simulink model "SWC_HALIN_type"  (R2021b)
settings: Solver=FixedStepDiscrete  StartTime=0.0  StopTime=10.0  FixedStep=0.005  RelTol=1e-3
undefined symbols (not defined in the file): FALSE, R_WDGCDD_CSOP_Call_Watchdog, R_WDGCDD_CSOP_Call_WDG_AppStart, TRUE
libraries: halin x1
settings Model: DataDictionary=APPTypes.sldd  Creator=FVT23010  LastModifiedBy=FVT23010
settings DataIOCC: SaveFormat=StructureWithTime
settings OptimizationCC: DefaultParameterBehavior=Inlined  EnhancedBackFolding=on  PassReuseOutputArgsAs=Individual arguments  ZeroExternalMemoryAtStartup=off  ZeroInternalMemoryAtStartup=off  OptimizeBlockOrder=speed  DifferentSizesBufferReuse=on  OptimizationCustomize=off  EfficientTunableParamExpr=on
settings DebuggingCC: ParameterTunabilityLossMsg=error
settings ModelReferenceCC: ModelReferenceNumInstancesAllowed=Single
settings SFSimCC: MATLABDynamicMemAlloc=off
settings RTWCC: Description=AUTOSAR  SystemTargetFile=autosar.tlc  GenCodeOnly=on  TemplateMakefile=ert_default_tmf
settings CodeAppCC: ForceParamTrailComments=on  IgnoreCustomStorageClasses=off  OperatorAnnotations=on  SimulinkDataObjDesc=on  SFDataObjDesc=on  InsertBlockDesc=on
settings STFCustomTargetCC: TargetLangStandard=C99 (ISO)  MultiwordLength=256  ParMdlRefBuildCompliant=on  CompOptLevelCompliant=on  IncludeMdlTerminateFcn=off  CombineOutputUpdateFcns=on  SuppressErrorStatus=on  ERTCustomFileBanners=on  SupportNonFinite=off  SupportComplex=off  SupportContinuousTime=off  SupportNonInlinedSFcns=off  RemoveResetFunc=on  MATLABClassNameForMDSCustomization=Simulink.SoftwareTarget.ERTCustomization  AutosarCompliant=on  GRTInterface=off  UseToolchainInfoCompliant=on  LookupTableObjectStructAxisOrder=2,1,3,4,...  LUTObjectStructOrderEvenSpacing=Size,Table,Breakpoints  SystemTargetFile=autosar.tlc
settings ERTTargetCC: TargetLangStandard=C99 (ISO)  ConcurrentExecutionCompliant=off  IncludeMdlTerminateFcn=off  SuppressErrorStatus=on  SupportNonFinite=off  SupportComplex=off  ModelStepFunctionPrototypeControlCompliant=off  CPPClassGenCompliant=off  AutosarCompliant=on  LookupTableObjectStructAxisOrder=2,1,3,4,...  LUTObjectStructOrderEvenSpacing=Size,Table,Breakpoints  InlinedParameterPlacement=NonHierarchical  ERTCustomFileTemplate=example_file_process.tlc

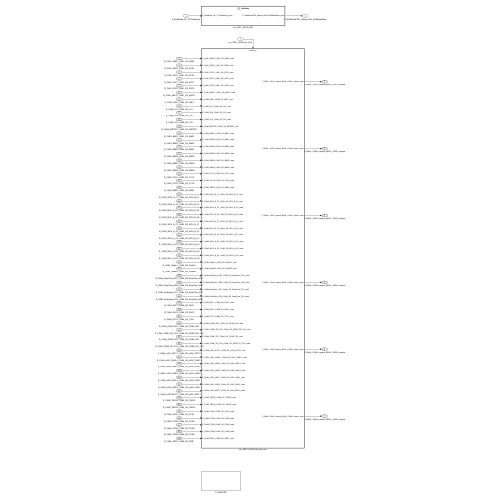
[thumbnail: Simulink's stored preview of the top-level diagram]
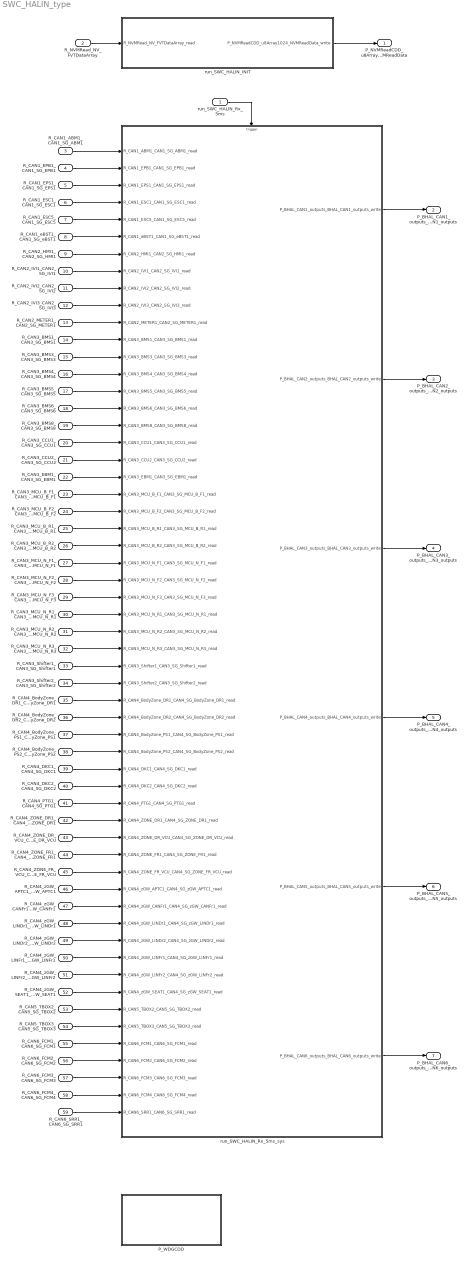
== system SWC_HALIN_type ==
  run_SWC_HALIN_Rx_5ms : Inport  SampleTime=0.005  OutputFunctionCall=on
  R_NVMRead_NV_FVTDataArray : Inport  Port=2  OutDataTypeStr=uint8  PortDimensions=1024
  R_CAN1_ABM1_CAN1_SG_ABM1 : Inport  Port=3  OutDataTypeStr=Bus: DT_CAN1_SG_ABM1  PortDimensions=1  BusOutputAsStruct=on
  R_CAN1_EPB1_CAN1_SG_EPB1 : Inport  Port=4  OutDataTypeStr=Bus: DT_CAN1_SG_EPB1  PortDimensions=1  BusOutputAsStruct=on
  R_CAN1_EPS1_CAN1_SG_EPS1 : Inport  Port=5  OutDataTypeStr=Bus: DT_CAN1_SG_EPS1  PortDimensions=1  BusOutputAsStruct=on
  R_CAN1_ESC1_CAN1_SG_ESC1 : Inport  Port=6  OutDataTypeStr=Bus: DT_CAN1_SG_ESC1  PortDimensions=1  BusOutputAsStruct=on
  R_CAN1_ESC5_CAN1_SG_ESC5 : Inport  Port=7  OutDataTypeStr=Bus: DT_CAN1_SG_ESC5  PortDimensions=1  BusOutputAsStruct=on
  R_CAN1_eBST1_CAN1_SG_eBST1 : Inport  Port=8  OutDataTypeStr=Bus: DT_CAN1_SG_eBST1  PortDimensions=1  BusOutputAsStruct=on
  R_CAN2_HMI1_CAN2_SG_HMI1 : Inport  Port=9  OutDataTypeStr=Bus: DT_CAN2_SG_HMI1  PortDimensions=1  BusOutputAsStruct=on
  R_CAN2_IVI1_CAN2_SG_IVI1 : Inport  Port=10  OutDataTypeStr=Bus: DT_CAN2_SG_IVI1  PortDimensions=1  BusOutputAsStruct=on
  R_CAN2_IVI2_CAN2_SG_IVI2 : Inport  Port=11  OutDataTypeStr=Bus: DT_CAN2_SG_IVI2  PortDimensions=1  BusOutputAsStruct=on
  R_CAN2_IVI3_CAN2_SG_IVI3 : Inport  Port=12  OutDataTypeStr=Bus: DT_CAN2_SG_IVI3  PortDimensions=1  BusOutputAsStruct=on
  R_CAN2_METER1_CAN2_SG_METER1 : Inport  Port=13  OutDataTypeStr=Bus: DT_CAN2_SG_METER1  PortDimensions=1  BusOutputAsStruct=on
  R_CAN3_BMS1_CAN3_SG_BMS1 : Inport  Port=14  OutDataTypeStr=Bus: DT_CAN3_SG_BMS1  PortDimensions=1  BusOutputAsStruct=on
  R_CAN3_BMS3_CAN3_SG_BMS3 : Inport  Port=15  OutDataTypeStr=Bus: DT_CAN3_SG_BMS3  PortDimensions=1  BusOutputAsStruct=on
  R_CAN3_BMS4_CAN3_SG_BMS4 : Inport  Port=16  OutDataTypeStr=Bus: DT_CAN3_SG_BMS4  PortDimensions=1  BusOutputAsStruct=on
  R_CAN3_BMS5_CAN3_SG_BMS5 : Inport  Port=17  OutDataTypeStr=Bus: DT_CAN3_SG_BMS5  PortDimensions=1  BusOutputAsStruct=on
  R_CAN3_BMS6_CAN3_SG_BMS6 : Inport  Port=18  OutDataTypeStr=Bus: DT_CAN3_SG_BMS6  PortDimensions=1  BusOutputAsStruct=on
  R_CAN3_BMS8_CAN3_SG_BMS8 : Inport  Port=19  OutDataTypeStr=Bus: DT_CAN3_SG_BMS8  PortDimensions=1  BusOutputAsStruct=on
  R_CAN3_CCU1_CAN3_SG_CCU1 : Inport  Port=20  OutDataTypeStr=Bus: DT_CAN3_SG_CCU1  PortDimensions=1  BusOutputAsStruct=on
  R_CAN3_CCU2_CAN3_SG_CCU2 : Inport  Port=21  OutDataTypeStr=Bus: DT_CAN3_SG_CCU2  PortDimensions=1  BusOutputAsStruct=on
  R_CAN3_EBM1_CAN3_SG_EBM1 : Inport  Port=22  OutDataTypeStr=Bus: DT_CAN3_SG_EBM1  PortDimensions=1  BusOutputAsStruct=on
  R_CAN3_MCU_B_F1_CAN3_SG_MCU_B_F1 : Inport  Port=23  OutDataTypeStr=Bus: DT_CAN3_SG_MCU_B_F1  PortDimensions=1  BusOutputAsStruct=on
  R_CAN3_MCU_B_F2_CAN3_SG_MCU_B_F2 : Inport  Port=24  OutDataTypeStr=Bus: DT_CAN3_SG_MCU_B_F2  PortDimensions=1  BusOutputAsStruct=on
  R_CAN3_MCU_B_R1_CAN3_SG_MCU_B_R1 : Inport  Port=25  OutDataTypeStr=Bus: DT_CAN3_SG_MCU_B_R1  PortDimensions=1  BusOutputAsStruct=on
  R_CAN3_MCU_B_R2_CAN3_SG_MCU_B_R2 : Inport  Port=26  OutDataTypeStr=Bus: DT_CAN3_SG_MCU_B_R2  PortDimensions=1  BusOutputAsStruct=on
  R_CAN3_MCU_N_F1_CAN3_SG_MCU_N_F1 : Inport  Port=27  OutDataTypeStr=Bus: DT_CAN3_SG_MCU_N_F1  PortDimensions=1  BusOutputAsStruct=on
  R_CAN3_MCU_N_F2_CAN3_SG_MCU_N_F2 : Inport  Port=28  OutDataTypeStr=Bus: DT_CAN3_SG_MCU_N_F2  PortDimensions=1  BusOutputAsStruct=on
  R_CAN3_MCU_N_F3_CAN3_SG_MCU_N_F3 : Inport  Port=29  OutDataTypeStr=Bus: DT_CAN3_SG_MCU_N_F3  PortDimensions=1  BusOutputAsStruct=on
  R_CAN3_MCU_N_R1_CAN3_SG_MCU_N_R1 : Inport  Port=30  OutDataTypeStr=Bus: DT_CAN3_SG_MCU_N_R1  PortDimensions=1  BusOutputAsStruct=on
  R_CAN3_MCU_N_R2_CAN3_SG_MCU_N_R2 : Inport  Port=31  OutDataTypeStr=Bus: DT_CAN3_SG_MCU_N_R2  PortDimensions=1  BusOutputAsStruct=on
  R_CAN3_MCU_N_R3_CAN3_SG_MCU_N_R3 : Inport  Port=32  OutDataTypeStr=Bus: DT_CAN3_SG_MCU_N_R3  PortDimensions=1  BusOutputAsStruct=on
  R_CAN3_Shifter1_CAN3_SG_Shifter1 : Inport  Port=33  OutDataTypeStr=Bus: DT_CAN3_SG_Shifter1  PortDimensions=1  BusOutputAsStruct=on
  R_CAN3_Shifter2_CAN3_SG_Shifter2 : Inport  Port=34  OutDataTypeStr=Bus: DT_CAN3_SG_Shifter2  PortDimensions=1  BusOutputAsStruct=on
  R_CAN4_BodyZone_DR1_CAN4_SG_BodyZone_DR1 : Inport  Port=35  OutDataTypeStr=Bus: DT_CAN4_SG_BodyZone_DR1  PortDimensions=1  BusOutputAsStruct=on
  R_CAN4_BodyZone_DR2_CAN4_SG_BodyZone_DR2 : Inport  Port=36  OutDataTypeStr=Bus: DT_CAN4_SG_BodyZone_DR2  PortDimensions=1  BusOutputAsStruct=on
  R_CAN4_BodyZone_PS1_CAN4_SG_BodyZone_PS1 : Inport  Port=37  OutDataTypeStr=Bus: DT_CAN4_SG_BodyZone_PS1  PortDimensions=1  BusOutputAsStruct=on
  R_CAN4_BodyZone_PS2_CAN4_SG_BodyZone_PS2 : Inport  Port=38  OutDataTypeStr=Bus: DT_CAN4_SG_BodyZone_PS2  PortDimensions=1  BusOutputAsStruct=on
  R_CAN4_DKC1_CAN4_SG_DKC1 : Inport  Port=39  OutDataTypeStr=Bus: DT_CAN4_SG_DKC1  PortDimensions=1  BusOutputAsStruct=on
  R_CAN4_DKC2_CAN4_SG_DKC2 : Inport  Port=40  OutDataTypeStr=Bus: DT_CAN4_SG_DKC2  PortDimensions=1  BusOutputAsStruct=on
  R_CAN4_PTG1_CAN4_SG_PTG1 : Inport  Port=41  OutDataTypeStr=Bus: DT_CAN4_SG_PTG1  PortDimensions=1  BusOutputAsStruct=on
  R_CAN4_ZONE_DR1_CAN4_SG_ZONE_DR1 : Inport  Port=42  OutDataTypeStr=Bus: DT_CAN4_SG_ZONE_DR1  PortDimensions=1  BusOutputAsStruct=on
  R_CAN4_ZONE_DR_VCU_CAN4_SG_ZONE_DR_VCU : Inport  Port=43  OutDataTypeStr=Bus: DT_CAN4_SG_ZONE_DR_VCU  PortDimensions=1  BusOutputAsStruct=on
  R_CAN4_ZONE_FR1_CAN4_SG_ZONE_FR1 : Inport  Port=44  OutDataTypeStr=Bus: DT_CAN4_SG_ZONE_FR1  PortDimensions=1  BusOutputAsStruct=on
  R_CAN4_ZONE_FR_VCU_CAN4_SG_ZONE_FR_VCU : Inport  Port=45  OutDataTypeStr=Bus: DT_CAN4_SG_ZONE_FR_VCU  PortDimensions=1  BusOutputAsStruct=on
  R_CAN4_zGW_APTC1_CAN4_SG_zGW_APTC1 : Inport  Port=46  OutDataTypeStr=Bus: DT_CAN4_SG_zGW_APTC1  PortDimensions=1  BusOutputAsStruct=on
  R_CAN4_zGW_CANFr1_CAN4_SG_zGW_CANFr1 : Inport  Port=47  OutDataTypeStr=Bus: DT_CAN4_SG_zGW_CANFr1  PortDimensions=1  BusOutputAsStruct=on
  R_CAN4_zGW_LINDr1_CAN4_SG_zGW_LINDr1 : Inport  Port=48  OutDataTypeStr=Bus: DT_CAN4_SG_zGW_LINDr1  PortDimensions=1  BusOutputAsStruct=on
  R_CAN4_zGW_LINDr2_CAN4_SG_zGW_LINDr2 : Inport  Port=49  OutDataTypeStr=Bus: DT_CAN4_SG_zGW_LINDr2  PortDimensions=1  BusOutputAsStruct=on
  R_CAN4_zGW_LINFr1_CAN4_SG_zGW_LINFr1 : Inport  Port=50  OutDataTypeStr=Bus: DT_CAN4_SG_zGW_LINFr1  PortDimensions=1  BusOutputAsStruct=on
  R_CAN4_zGW_LINFr2_CAN4_SG_zGW_LINFr2 : Inport  Port=51  OutDataTypeStr=Bus: DT_CAN4_SG_zGW_LINFr2  PortDimensions=1  BusOutputAsStruct=on
  R_CAN4_zGW_SEAT1_CAN4_SG_zGW_SEAT1 : Inport  Port=52  OutDataTypeStr=Bus: DT_CAN4_SG_zGW_SEAT1  PortDimensions=1  BusOutputAsStruct=on
  R_CAN5_TBOX2_CAN5_SG_TBOX2 : Inport  Port=53  OutDataTypeStr=Bus: DT_CAN5_SG_TBOX2  PortDimensions=1  BusOutputAsStruct=on
  R_CAN5_TBOX3_CAN5_SG_TBOX3 : Inport  Port=54  OutDataTypeStr=Bus: DT_CAN5_SG_TBOX3  PortDimensions=1  BusOutputAsStruct=on
  R_CAN6_FCM1_CAN6_SG_FCM1 : Inport  Port=55  OutDataTypeStr=Bus: DT_CAN6_SG_FCM1  PortDimensions=1  BusOutputAsStruct=on
  R_CAN6_FCM2_CAN6_SG_FCM2 : Inport  Port=56  OutDataTypeStr=Bus: DT_CAN6_SG_FCM2  PortDimensions=1  BusOutputAsStruct=on
  R_CAN6_FCM3_CAN6_SG_FCM3 : Inport  Port=57  OutDataTypeStr=Bus: DT_CAN6_SG_FCM3  PortDimensions=1  BusOutputAsStruct=on
  R_CAN6_FCM4_CAN6_SG_FCM4 : Inport  Port=58  OutDataTypeStr=Bus: DT_CAN6_SG_FCM4  PortDimensions=1  BusOutputAsStruct=on
  R_CAN6_SRR1_CAN6_SG_SRR1 : Inport  Port=59  OutDataTypeStr=Bus: DT_CAN6_SG_SRR1  PortDimensions=1  BusOutputAsStruct=on
  P_WDGCDD : Subsystem
  run_SWC_HALIN_INIT : Subsystem
  run_SWC_HALIN_Rx_5ms_sys : Subsystem
  P_NVMReadCDD_u8Array1024_NVMReadData : Outport  OutDataTypeStr=uint8  PortDimensions=1024
  P_BHAL_CAN1_outputs_BHAL_CAN1_outputs : Outport  Port=2  OutDataTypeStr=Bus: BHAL_CAN1_outputs  PortDimensions=1  BusOutputAsStruct=on
  P_BHAL_CAN2_outputs_BHAL_CAN2_outputs : Outport  Port=3  OutDataTypeStr=Bus: BHAL_CAN2_outputs  PortDimensions=1  BusOutputAsStruct=on
  P_BHAL_CAN3_outputs_BHAL_CAN3_outputs : Outport  Port=4  OutDataTypeStr=Bus: BHAL_CAN3_outputs  PortDimensions=1  BusOutputAsStruct=on
  P_BHAL_CAN4_outputs_BHAL_CAN4_outputs : Outport  Port=5  OutDataTypeStr=Bus: BHAL_CAN4_outputs  PortDimensions=1  BusOutputAsStruct=on
  P_BHAL_CAN5_outputs_BHAL_CAN5_outputs : Outport  Port=6  OutDataTypeStr=Bus: BHAL_CAN5_outputs  PortDimensions=1  BusOutputAsStruct=on
  P_BHAL_CAN6_outputs_BHAL_CAN6_outputs : Outport  Port=7  OutDataTypeStr=Bus: BHAL_CAN6_outputs  PortDimensions=1  BusOutputAsStruct=on
  wires:
  R_NVMRead_NV_FVTDataArray/1 -> run_SWC_HALIN_INIT/1(R_NVMRead_NV_FVTDataArray_read)
  run_SWC_HALIN_INIT/1(P_NVMReadCDD_u8Array1024_NVMReadData_write) -> P_NVMReadCDD_u8Array1024_NVMReadData/1
  R_CAN1_ABM1_CAN1_SG_ABM1/1 -> run_SWC_HALIN_Rx_5ms_sys/1(R_CAN1_ABM1_CAN1_SG_ABM1_read)
  R_CAN1_EPB1_CAN1_SG_EPB1/1 -> run_SWC_HALIN_Rx_5ms_sys/2(R_CAN1_EPB1_CAN1_SG_EPB1_read)
  R_CAN1_EPS1_CAN1_SG_EPS1/1 -> run_SWC_HALIN_Rx_5ms_sys/3(R_CAN1_EPS1_CAN1_SG_EPS1_read)
  R_CAN1_ESC1_CAN1_SG_ESC1/1 -> run_SWC_HALIN_Rx_5ms_sys/4(R_CAN1_ESC1_CAN1_SG_ESC1_read)
  R_CAN1_ESC5_CAN1_SG_ESC5/1 -> run_SWC_HALIN_Rx_5ms_sys/5(R_CAN1_ESC5_CAN1_SG_ESC5_read)
  R_CAN1_eBST1_CAN1_SG_eBST1/1 -> run_SWC_HALIN_Rx_5ms_sys/6(R_CAN1_eBST1_CAN1_SG_eBST1_read)
  R_CAN2_HMI1_CAN2_SG_HMI1/1 -> run_SWC_HALIN_Rx_5ms_sys/7(R_CAN2_HMI1_CAN2_SG_HMI1_read)
  R_CAN2_IVI1_CAN2_SG_IVI1/1 -> run_SWC_HALIN_Rx_5ms_sys/8(R_CAN2_IVI1_CAN2_SG_IVI1_read)
  R_CAN2_IVI2_CAN2_SG_IVI2/1 -> run_SWC_HALIN_Rx_5ms_sys/9(R_CAN2_IVI2_CAN2_SG_IVI2_read)
  R_CAN2_IVI3_CAN2_SG_IVI3/1 -> run_SWC_HALIN_Rx_5ms_sys/10(R_CAN2_IVI3_CAN2_SG_IVI3_read)
  R_CAN2_METER1_CAN2_SG_METER1/1 -> run_SWC_HALIN_Rx_5ms_sys/11(R_CAN2_METER1_CAN2_SG_METER1_read)
  R_CAN3_BMS1_CAN3_SG_BMS1/1 -> run_SWC_HALIN_Rx_5ms_sys/12(R_CAN3_BMS1_CAN3_SG_BMS1_read)
  R_CAN3_BMS3_CAN3_SG_BMS3/1 -> run_SWC_HALIN_Rx_5ms_sys/13(R_CAN3_BMS3_CAN3_SG_BMS3_read)
  R_CAN3_BMS4_CAN3_SG_BMS4/1 -> run_SWC_HALIN_Rx_5ms_sys/14(R_CAN3_BMS4_CAN3_SG_BMS4_read)
  R_CAN3_BMS5_CAN3_SG_BMS5/1 -> run_SWC_HALIN_Rx_5ms_sys/15(R_CAN3_BMS5_CAN3_SG_BMS5_read)
  R_CAN3_BMS6_CAN3_SG_BMS6/1 -> run_SWC_HALIN_Rx_5ms_sys/16(R_CAN3_BMS6_CAN3_SG_BMS6_read)
  R_CAN3_BMS8_CAN3_SG_BMS8/1 -> run_SWC_HALIN_Rx_5ms_sys/17(R_CAN3_BMS8_CAN3_SG_BMS8_read)
  R_CAN3_CCU1_CAN3_SG_CCU1/1 -> run_SWC_HALIN_Rx_5ms_sys/18(R_CAN3_CCU1_CAN3_SG_CCU1_read)
  R_CAN3_CCU2_CAN3_SG_CCU2/1 -> run_SWC_HALIN_Rx_5ms_sys/19(R_CAN3_CCU2_CAN3_SG_CCU2_read)
  R_CAN3_EBM1_CAN3_SG_EBM1/1 -> run_SWC_HALIN_Rx_5ms_sys/20(R_CAN3_EBM1_CAN3_SG_EBM1_read)
  R_CAN3_MCU_B_F1_CAN3_SG_MCU_B_F1/1 -> run_SWC_HALIN_Rx_5ms_sys/21(R_CAN3_MCU_B_F1_CAN3_SG_MCU_B_F1_read)
  R_CAN3_MCU_B_F2_CAN3_SG_MCU_B_F2/1 -> run_SWC_HALIN_Rx_5ms_sys/22(R_CAN3_MCU_B_F2_CAN3_SG_MCU_B_F2_read)
  R_CAN3_MCU_B_R1_CAN3_SG_MCU_B_R1/1 -> run_SWC_HALIN_Rx_5ms_sys/23(R_CAN3_MCU_B_R1_CAN3_SG_MCU_B_R1_read)
  R_CAN3_MCU_B_R2_CAN3_SG_MCU_B_R2/1 -> run_SWC_HALIN_Rx_5ms_sys/24(R_CAN3_MCU_B_R2_CAN3_SG_MCU_B_R2_read)
  R_CAN3_MCU_N_F1_CAN3_SG_MCU_N_F1/1 -> run_SWC_HALIN_Rx_5ms_sys/25(R_CAN3_MCU_N_F1_CAN3_SG_MCU_N_F1_read)
  R_CAN3_MCU_N_F2_CAN3_SG_MCU_N_F2/1 -> run_SWC_HALIN_Rx_5ms_sys/26(R_CAN3_MCU_N_F2_CAN3_SG_MCU_N_F2_read)
  R_CAN3_MCU_N_F3_CAN3_SG_MCU_N_F3/1 -> run_SWC_HALIN_Rx_5ms_sys/27(R_CAN3_MCU_N_F3_CAN3_SG_MCU_N_F3_read)
  R_CAN3_MCU_N_R1_CAN3_SG_MCU_N_R1/1 -> run_SWC_HALIN_Rx_5ms_sys/28(R_CAN3_MCU_N_R1_CAN3_SG_MCU_N_R1_read)
  R_CAN3_MCU_N_R2_CAN3_SG_MCU_N_R2/1 -> run_SWC_HALIN_Rx_5ms_sys/29(R_CAN3_MCU_N_R2_CAN3_SG_MCU_N_R2_read)
  R_CAN3_MCU_N_R3_CAN3_SG_MCU_N_R3/1 -> run_SWC_HALIN_Rx_5ms_sys/30(R_CAN3_MCU_N_R3_CAN3_SG_MCU_N_R3_read)
  R_CAN3_Shifter1_CAN3_SG_Shifter1/1 -> run_SWC_HALIN_Rx_5ms_sys/31(R_CAN3_Shifter1_CAN3_SG_Shifter1_read)
  R_CAN3_Shifter2_CAN3_SG_Shifter2/1 -> run_SWC_HALIN_Rx_5ms_sys/32(R_CAN3_Shifter2_CAN3_SG_Shifter2_read)
  R_CAN4_BodyZone_DR1_CAN4_SG_BodyZone_DR1/1 -> run_SWC_HALIN_Rx_5ms_sys/33(R_CAN4_BodyZone_DR1_CAN4_SG_BodyZone_DR1_read)
  R_CAN4_BodyZone_DR2_CAN4_SG_BodyZone_DR2/1 -> run_SWC_HALIN_Rx_5ms_sys/34(R_CAN4_BodyZone_DR2_CAN4_SG_BodyZone_DR2_read)
  R_CAN4_BodyZone_PS1_CAN4_SG_BodyZone_PS1/1 -> run_SWC_HALIN_Rx_5ms_sys/35(R_CAN4_BodyZone_PS1_CAN4_SG_BodyZone_PS1_read)
  R_CAN4_BodyZone_PS2_CAN4_SG_BodyZone_PS2/1 -> run_SWC_HALIN_Rx_5ms_sys/36(R_CAN4_BodyZone_PS2_CAN4_SG_BodyZone_PS2_read)
  R_CAN4_DKC1_CAN4_SG_DKC1/1 -> run_SWC_HALIN_Rx_5ms_sys/37(R_CAN4_DKC1_CAN4_SG_DKC1_read)
  R_CAN4_DKC2_CAN4_SG_DKC2/1 -> run_SWC_HALIN_Rx_5ms_sys/38(R_CAN4_DKC2_CAN4_SG_DKC2_read)
  R_CAN4_PTG1_CAN4_SG_PTG1/1 -> run_SWC_HALIN_Rx_5ms_sys/39(R_CAN4_PTG1_CAN4_SG_PTG1_read)
  R_CAN4_ZONE_DR1_CAN4_SG_ZONE_DR1/1 -> run_SWC_HALIN_Rx_5ms_sys/40(R_CAN4_ZONE_DR1_CAN4_SG_ZONE_DR1_read)
  R_CAN4_ZONE_DR_VCU_CAN4_SG_ZONE_DR_VCU/1 -> run_SWC_HALIN_Rx_5ms_sys/41(R_CAN4_ZONE_DR_VCU_CAN4_SG_ZONE_DR_VCU_read)
  R_CAN4_ZONE_FR1_CAN4_SG_ZONE_FR1/1 -> run_SWC_HALIN_Rx_5ms_sys/42(R_CAN4_ZONE_FR1_CAN4_SG_ZONE_FR1_read)
  R_CAN4_ZONE_FR_VCU_CAN4_SG_ZONE_FR_VCU/1 -> run_SWC_HALIN_Rx_5ms_sys/43(R_CAN4_ZONE_FR_VCU_CAN4_SG_ZONE_FR_VCU_read)
  R_CAN4_zGW_APTC1_CAN4_SG_zGW_APTC1/1 -> run_SWC_HALIN_Rx_5ms_sys/44(R_CAN4_zGW_APTC1_CAN4_SG_zGW_APTC1_read)
  R_CAN4_zGW_CANFr1_CAN4_SG_zGW_CANFr1/1 -> run_SWC_HALIN_Rx_5ms_sys/45(R_CAN4_zGW_CANFr1_CAN4_SG_zGW_CANFr1_read)
  R_CAN4_zGW_LINDr1_CAN4_SG_zGW_LINDr1/1 -> run_SWC_HALIN_Rx_5ms_sys/46(R_CAN4_zGW_LINDr1_CAN4_SG_zGW_LINDr1_read)
  R_CAN4_zGW_LINDr2_CAN4_SG_zGW_LINDr2/1 -> run_SWC_HALIN_Rx_5ms_sys/47(R_CAN4_zGW_LINDr2_CAN4_SG_zGW_LINDr2_read)
  R_CAN4_zGW_LINFr1_CAN4_SG_zGW_LINFr1/1 -> run_SWC_HALIN_Rx_5ms_sys/48(R_CAN4_zGW_LINFr1_CAN4_SG_zGW_LINFr1_read)
  R_CAN4_zGW_LINFr2_CAN4_SG_zGW_LINFr2/1 -> run_SWC_HALIN_Rx_5ms_sys/49(R_CAN4_zGW_LINFr2_CAN4_SG_zGW_LINFr2_read)
  R_CAN4_zGW_SEAT1_CAN4_SG_zGW_SEAT1/1 -> run_SWC_HALIN_Rx_5ms_sys/50(R_CAN4_zGW_SEAT1_CAN4_SG_zGW_SEAT1_read)
  R_CAN5_TBOX2_CAN5_SG_TBOX2/1 -> run_SWC_HALIN_Rx_5ms_sys/51(R_CAN5_TBOX2_CAN5_SG_TBOX2_read)
  R_CAN5_TBOX3_CAN5_SG_TBOX3/1 -> run_SWC_HALIN_Rx_5ms_sys/52(R_CAN5_TBOX3_CAN5_SG_TBOX3_read)
  R_CAN6_FCM1_CAN6_SG_FCM1/1 -> run_SWC_HALIN_Rx_5ms_sys/53(R_CAN6_FCM1_CAN6_SG_FCM1_read)
  R_CAN6_FCM2_CAN6_SG_FCM2/1 -> run_SWC_HALIN_Rx_5ms_sys/54(R_CAN6_FCM2_CAN6_SG_FCM2_read)
  R_CAN6_FCM3_CAN6_SG_FCM3/1 -> run_SWC_HALIN_Rx_5ms_sys/55(R_CAN6_FCM3_CAN6_SG_FCM3_read)
  R_CAN6_FCM4_CAN6_SG_FCM4/1 -> run_SWC_HALIN_Rx_5ms_sys/56(R_CAN6_FCM4_CAN6_SG_FCM4_read)
  R_CAN6_SRR1_CAN6_SG_SRR1/1 -> run_SWC_HALIN_Rx_5ms_sys/57(R_CAN6_SRR1_CAN6_SG_SRR1_read)
  run_SWC_HALIN_Rx_5ms_sys/1(P_BHAL_CAN1_outputs_BHAL_CAN1_outputs_write) -> P_BHAL_CAN1_outputs_BHAL_CAN1_outputs/1
  run_SWC_HALIN_Rx_5ms_sys/2(P_BHAL_CAN2_outputs_BHAL_CAN2_outputs_write) -> P_BHAL_CAN2_outputs_BHAL_CAN2_outputs/1
  run_SWC_HALIN_Rx_5ms_sys/3(P_BHAL_CAN3_outputs_BHAL_CAN3_outputs_write) -> P_BHAL_CAN3_outputs_BHAL_CAN3_outputs/1
  run_SWC_HALIN_Rx_5ms_sys/4(P_BHAL_CAN4_outputs_BHAL_CAN4_outputs_write) -> P_BHAL_CAN4_outputs_BHAL_CAN4_outputs/1
  run_SWC_HALIN_Rx_5ms_sys/5(P_BHAL_CAN5_outputs_BHAL_CAN5_outputs_write) -> P_BHAL_CAN5_outputs_BHAL_CAN5_outputs/1
  run_SWC_HALIN_Rx_5ms_sys/6(P_BHAL_CAN6_outputs_BHAL_CAN6_outputs_write) -> P_BHAL_CAN6_outputs_BHAL_CAN6_outputs/1
  run_SWC_HALIN_Rx_5ms/1 -> run_SWC_HALIN_Rx_5ms_sys/Trigger

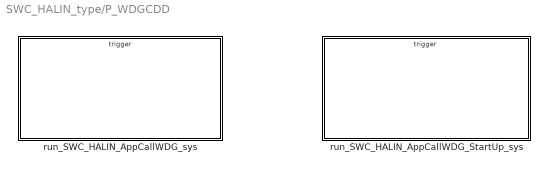
== system SWC_HALIN_type/P_WDGCDD ==
  run_SWC_HALIN_AppCallWDG_StartUp_sys : Subsystem
  run_SWC_HALIN_AppCallWDG_sys : Subsystem

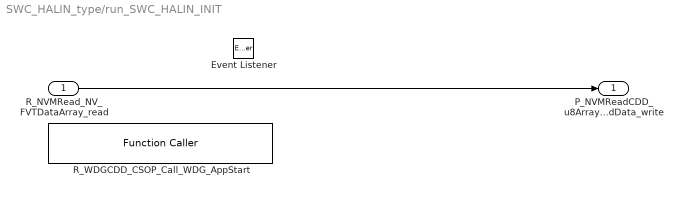
== system SWC_HALIN_type/run_SWC_HALIN_INIT ==
  R_NVMRead_NV_FVTDataArray_read : Inport
  Event Listener : EventListener  EventName=reset
  R_WDGCDD_CSOP_Call_WDG_AppStart : FunctionCaller  FunctionPrototype=R_WDGCDD_CSOP_Call_WDG_AppStart()
  P_NVMReadCDD_u8Array1024_NVMReadData_write : Outport
  wires:
  R_NVMRead_NV_FVTDataArray_read/1 -> P_NVMReadCDD_u8Array1024_NVMReadData_write/1

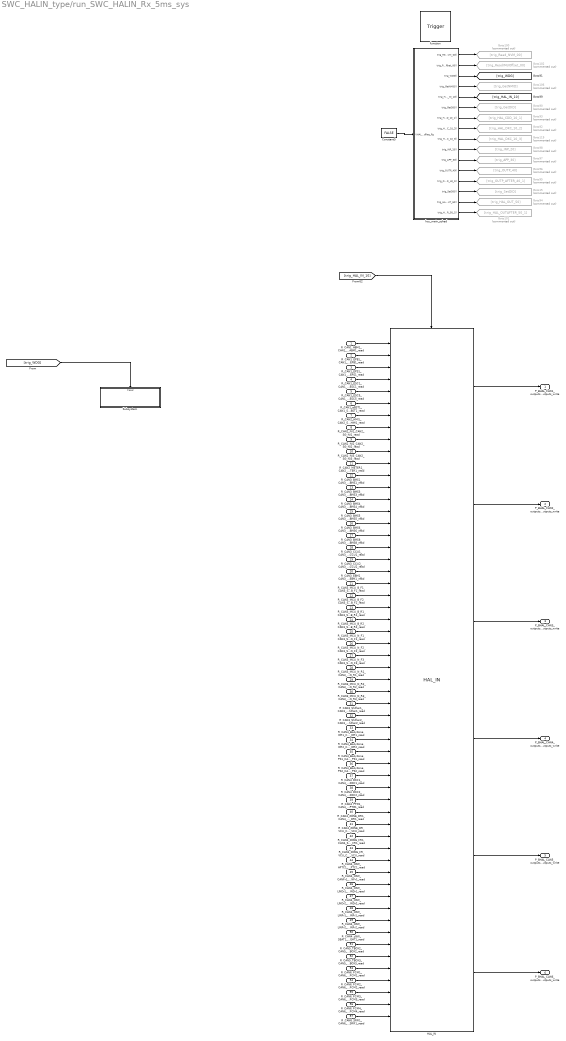
== system SWC_HALIN_type/run_SWC_HALIN_Rx_5ms_sys ==
  R_CAN1_ABM1_CAN1_SG_ABM1_read : Inport
  R_CAN1_EPB1_CAN1_SG_EPB1_read : Inport  Port=2
  R_CAN1_EPS1_CAN1_SG_EPS1_read : Inport  Port=3
  R_CAN1_ESC1_CAN1_SG_ESC1_read : Inport  Port=4
  R_CAN1_ESC5_CAN1_SG_ESC5_read : Inport  Port=5
  R_CAN1_eBST1_CAN1_SG_eBST1_read : Inport  Port=6
  R_CAN2_HMI1_CAN2_SG_HMI1_read : Inport  Port=7
  R_CAN2_IVI1_CAN2_SG_IVI1_read : Inport  Port=8
  R_CAN2_IVI2_CAN2_SG_IVI2_read : Inport  Port=9
  R_CAN2_IVI3_CAN2_SG_IVI3_read : Inport  Port=10
  R_CAN2_METER1_CAN2_SG_METER1_read : Inport  Port=11
  R_CAN3_BMS1_CAN3_SG_BMS1_read : Inport  Port=12
  R_CAN3_BMS3_CAN3_SG_BMS3_read : Inport  Port=13
  R_CAN3_BMS4_CAN3_SG_BMS4_read : Inport  Port=14
  R_CAN3_BMS5_CAN3_SG_BMS5_read : Inport  Port=15
  R_CAN3_BMS6_CAN3_SG_BMS6_read : Inport  Port=16
  R_CAN3_BMS8_CAN3_SG_BMS8_read : Inport  Port=17
  R_CAN3_CCU1_CAN3_SG_CCU1_read : Inport  Port=18
  R_CAN3_CCU2_CAN3_SG_CCU2_read : Inport  Port=19
  R_CAN3_EBM1_CAN3_SG_EBM1_read : Inport  Port=20
  R_CAN3_MCU_B_F1_CAN3_SG_MCU_B_F1_read : Inport  Port=21
  R_CAN3_MCU_B_F2_CAN3_SG_MCU_B_F2_read : Inport  Port=22
  R_CAN3_MCU_B_R1_CAN3_SG_MCU_B_R1_read : Inport  Port=23
  R_CAN3_MCU_B_R2_CAN3_SG_MCU_B_R2_read : Inport  Port=24
  R_CAN3_MCU_N_F1_CAN3_SG_MCU_N_F1_read : Inport  Port=25
  R_CAN3_MCU_N_F2_CAN3_SG_MCU_N_F2_read : Inport  Port=26
  R_CAN3_MCU_N_F3_CAN3_SG_MCU_N_F3_read : Inport  Port=27
  R_CAN3_MCU_N_R1_CAN3_SG_MCU_N_R1_read : Inport  Port=28
  R_CAN3_MCU_N_R2_CAN3_SG_MCU_N_R2_read : Inport  Port=29
  R_CAN3_MCU_N_R3_CAN3_SG_MCU_N_R3_read : Inport  Port=30
  R_CAN3_Shifter1_CAN3_SG_Shifter1_read : Inport  Port=31
  R_CAN3_Shifter2_CAN3_SG_Shifter2_read : Inport  Port=32
  R_CAN4_BodyZone_DR1_CAN4_SG_BodyZone_DR1_read : Inport  Port=33
  R_CAN4_BodyZone_DR2_CAN4_SG_BodyZone_DR2_read : Inport  Port=34
  R_CAN4_BodyZone_PS1_CAN4_SG_BodyZone_PS1_read : Inport  Port=35
  R_CAN4_BodyZone_PS2_CAN4_SG_BodyZone_PS2_read : Inport  Port=36
  R_CAN4_DKC1_CAN4_SG_DKC1_read : Inport  Port=37
  R_CAN4_DKC2_CAN4_SG_DKC2_read : Inport  Port=38
  R_CAN4_PTG1_CAN4_SG_PTG1_read : Inport  Port=39
  R_CAN4_ZONE_DR1_CAN4_SG_ZONE_DR1_read : Inport  Port=40
  R_CAN4_ZONE_DR_VCU_CAN4_SG_ZONE_DR_VCU_read : Inport  Port=41
  R_CAN4_ZONE_FR1_CAN4_SG_ZONE_FR1_read : Inport  Port=42
  R_CAN4_ZONE_FR_VCU_CAN4_SG_ZONE_FR_VCU_read : Inport  Port=43
  R_CAN4_zGW_APTC1_CAN4_SG_zGW_APTC1_read : Inport  Port=44
  R_CAN4_zGW_CANFr1_CAN4_SG_zGW_CANFr1_read : Inport  Port=45
  R_CAN4_zGW_LINDr1_CAN4_SG_zGW_LINDr1_read : Inport  Port=46
  R_CAN4_zGW_LINDr2_CAN4_SG_zGW_LINDr2_read : Inport  Port=47
  R_CAN4_zGW_LINFr1_CAN4_SG_zGW_LINFr1_read : Inport  Port=48
  R_CAN4_zGW_LINFr2_CAN4_SG_zGW_LINFr2_read : Inport  Port=49
  R_CAN4_zGW_SEAT1_CAN4_SG_zGW_SEAT1_read : Inport  Port=50
  R_CAN5_TBOX2_CAN5_SG_TBOX2_read : Inport  Port=51
  R_CAN5_TBOX3_CAN5_SG_TBOX3_read : Inport  Port=52
  R_CAN6_FCM1_CAN6_SG_FCM1_read : Inport  Port=53
  R_CAN6_FCM2_CAN6_SG_FCM2_read : Inport  Port=54
  R_CAN6_FCM3_CAN6_SG_FCM3_read : Inport  Port=55
  R_CAN6_FCM4_CAN6_SG_FCM4_read : Inport  Port=56
  R_CAN6_SRR1_CAN6_SG_SRR1_read : Inport  Port=57
  function : TriggerPort  TriggerType=function-call  VariantControl=(inherit)  SampleTimeType=periodic  SampleTime=-1
  Constant5 : Constant  Value=FALSE
  Goto100 : Goto  Commented=on  GotoTag=trig_Read_NVM_00
  Goto101 : Goto  Commented=on  GotoTag=trig_HAL_OUTAFTER_50_1
  Goto102 : Goto  Commented=on  GotoTag=trig_ReadIMUOffset_00
  Goto106 : Goto  Commented=on  GotoTag=trig_GetNMID
  Goto119 : Goto  Commented=on  GotoTag=trig_HAL_DKC_10_3
  Goto15 : Goto  Commented=on  GotoTag=trig_SetDID
  Goto90 : Goto  Commented=on  GotoTag=trig_GetDID
  Goto92 : Goto  Commented=on  GotoTag=trig_HAL_DKC_10_2
  Goto93 : Goto  Commented=on  GotoTag=trig_HAL_CDD_10_1
  Goto94 : Goto  Commented=on  GotoTag=trig_HAL_OUT_50
  Goto95 : Goto  Commented=on  GotoTag=trig_OUTP_AFTER_40_1
  Goto96 : Goto  Commented=on  GotoTag=trig_OUTP_40
  Goto97 : Goto  Commented=on  GotoTag=trig_APP_30
  Goto98 : Goto  Commented=on  GotoTag=trig_INP_20
  HAL_IN : halin/HAL_IN  SystemSampleTime=-1  VariantActivationTime=update diagram  Latency=0  AutoFrameSizeCalculation=off
  Subsystem : Subsystem
  hcu_main_sched : Stateflow chart  TreatAsAtomicUnit=on
  P_BHAL_CAN1_outputs_BHAL_CAN1_outputs_write : Outport
  P_BHAL_CAN2_outputs_BHAL_CAN2_outputs_write : Outport  Port=2
  P_BHAL_CAN3_outputs_BHAL_CAN3_outputs_write : Outport  Port=3
  P_BHAL_CAN4_outputs_BHAL_CAN4_outputs_write : Outport  Port=4
  P_BHAL_CAN5_outputs_BHAL_CAN5_outputs_write : Outport  Port=5
  P_BHAL_CAN6_outputs_BHAL_CAN6_outputs_write : Outport  Port=6
  wires:
  hcu_main_sched/11(trig_APP_30()) -> Goto97/1
  hcu_main_sched/13(trig_OUTP_AFTER_40_1()) -> Goto95/1
  Constant5/1 -> hcu_main_sched/1(VHAL_FusionSchedReq_flg)
  hcu_main_sched/8(trig_HAL_DKC_10_2()) -> Goto92/1
  hcu_main_sched/10(trig_INP_20()) -> Goto98/1
  hcu_main_sched/16(trig_HAL_OUTAFTER_50_1()) -> Goto101/1
  hcu_main_sched/5(trig_HAL_IN_10()) -> [trig_HAL_IN_10]
  hcu_main_sched/3(trig_WDG()) -> [trig_WDG]
  hcu_main_sched/12(trig_OUTP_40()) -> Goto96/1
  hcu_main_sched/1(trig_Read_NVM_00()) -> Goto100/1
  hcu_main_sched/15(trig_HAL_OUT_50()) -> Goto94/1
  hcu_main_sched/9(trig_HAL_DKC_10_3()) -> Goto119/1
  hcu_main_sched/6(trig_GetDID()) -> Goto90/1
  hcu_main_sched/4(trig_GetNMID()) -> Goto106/1
  hcu_main_sched/7(trig_HAL_CDD_10_1()) -> Goto93/1
  hcu_main_sched/2(trig_ReadIMUOffset_00()) -> Goto102/1
  hcu_main_sched/14(trig_SetDID()) -> Goto15/1
  [trig_HAL_IN_10] -> HAL_IN/Trigger
  [trig_WDG] -> Subsystem/Trigger
  R_CAN1_ABM1_CAN1_SG_ABM1_read/1 -> HAL_IN/1
  R_CAN1_EPB1_CAN1_SG_EPB1_read/1 -> HAL_IN/2
  R_CAN1_EPS1_CAN1_SG_EPS1_read/1 -> HAL_IN/3
  R_CAN1_ESC1_CAN1_SG_ESC1_read/1 -> HAL_IN/4
  R_CAN1_ESC5_CAN1_SG_ESC5_read/1 -> HAL_IN/5
  R_CAN1_eBST1_CAN1_SG_eBST1_read/1 -> HAL_IN/6
  R_CAN2_HMI1_CAN2_SG_HMI1_read/1 -> HAL_IN/7
  R_CAN2_IVI1_CAN2_SG_IVI1_read/1 -> HAL_IN/8
  R_CAN2_IVI2_CAN2_SG_IVI2_read/1 -> HAL_IN/9
  R_CAN2_IVI3_CAN2_SG_IVI3_read/1 -> HAL_IN/10
  R_CAN2_METER1_CAN2_SG_METER1_read/1 -> HAL_IN/11
  R_CAN3_BMS1_CAN3_SG_BMS1_read/1 -> HAL_IN/12
  R_CAN3_BMS3_CAN3_SG_BMS3_read/1 -> HAL_IN/13
  R_CAN3_BMS4_CAN3_SG_BMS4_read/1 -> HAL_IN/14
  R_CAN3_BMS5_CAN3_SG_BMS5_read/1 -> HAL_IN/15
  R_CAN3_BMS6_CAN3_SG_BMS6_read/1 -> HAL_IN/16
  R_CAN3_BMS8_CAN3_SG_BMS8_read/1 -> HAL_IN/17
  R_CAN3_CCU1_CAN3_SG_CCU1_read/1 -> HAL_IN/18
  R_CAN3_CCU2_CAN3_SG_CCU2_read/1 -> HAL_IN/19
  R_CAN3_EBM1_CAN3_SG_EBM1_read/1 -> HAL_IN/20
  R_CAN3_MCU_B_F1_CAN3_SG_MCU_B_F1_read/1 -> HAL_IN/21
  R_CAN3_MCU_B_F2_CAN3_SG_MCU_B_F2_read/1 -> HAL_IN/22
  R_CAN3_MCU_B_R1_CAN3_SG_MCU_B_R1_read/1 -> HAL_IN/23
  R_CAN3_MCU_B_R2_CAN3_SG_MCU_B_R2_read/1 -> HAL_IN/24
  R_CAN3_MCU_N_F1_CAN3_SG_MCU_N_F1_read/1 -> HAL_IN/25
  R_CAN3_MCU_N_F2_CAN3_SG_MCU_N_F2_read/1 -> HAL_IN/26
  R_CAN3_MCU_N_F3_CAN3_SG_MCU_N_F3_read/1 -> HAL_IN/27
  R_CAN3_MCU_N_R1_CAN3_SG_MCU_N_R1_read/1 -> HAL_IN/28
  R_CAN3_MCU_N_R2_CAN3_SG_MCU_N_R2_read/1 -> HAL_IN/29
  R_CAN3_MCU_N_R3_CAN3_SG_MCU_N_R3_read/1 -> HAL_IN/30
  R_CAN3_Shifter1_CAN3_SG_Shifter1_read/1 -> HAL_IN/31
  R_CAN3_Shifter2_CAN3_SG_Shifter2_read/1 -> HAL_IN/32
  R_CAN4_BodyZone_DR1_CAN4_SG_BodyZone_DR1_read/1 -> HAL_IN/33
  R_CAN4_BodyZone_DR2_CAN4_SG_BodyZone_DR2_read/1 -> HAL_IN/34
  R_CAN4_BodyZone_PS1_CAN4_SG_BodyZone_PS1_read/1 -> HAL_IN/35
  R_CAN4_BodyZone_PS2_CAN4_SG_BodyZone_PS2_read/1 -> HAL_IN/36
  R_CAN4_DKC1_CAN4_SG_DKC1_read/1 -> HAL_IN/37
  R_CAN4_DKC2_CAN4_SG_DKC2_read/1 -> HAL_IN/38
  R_CAN4_PTG1_CAN4_SG_PTG1_read/1 -> HAL_IN/39
  R_CAN4_ZONE_DR1_CAN4_SG_ZONE_DR1_read/1 -> HAL_IN/40
  R_CAN4_ZONE_DR_VCU_CAN4_SG_ZONE_DR_VCU_read/1 -> HAL_IN/41
  R_CAN4_ZONE_FR1_CAN4_SG_ZONE_FR1_read/1 -> HAL_IN/42
  R_CAN4_ZONE_FR_VCU_CAN4_SG_ZONE_FR_VCU_read/1 -> HAL_IN/43
  R_CAN4_zGW_APTC1_CAN4_SG_zGW_APTC1_read/1 -> HAL_IN/44
  R_CAN4_zGW_CANFr1_CAN4_SG_zGW_CANFr1_read/1 -> HAL_IN/45
  R_CAN4_zGW_LINDr1_CAN4_SG_zGW_LINDr1_read/1 -> HAL_IN/46
  R_CAN4_zGW_LINDr2_CAN4_SG_zGW_LINDr2_read/1 -> HAL_IN/47
  R_CAN4_zGW_LINFr1_CAN4_SG_zGW_LINFr1_read/1 -> HAL_IN/48
  R_CAN4_zGW_LINFr2_CAN4_SG_zGW_LINFr2_read/1 -> HAL_IN/49
  R_CAN4_zGW_SEAT1_CAN4_SG_zGW_SEAT1_read/1 -> HAL_IN/50
  R_CAN5_TBOX2_CAN5_SG_TBOX2_read/1 -> HAL_IN/51
  R_CAN5_TBOX3_CAN5_SG_TBOX3_read/1 -> HAL_IN/52
  R_CAN6_FCM1_CAN6_SG_FCM1_read/1 -> HAL_IN/53
  R_CAN6_FCM2_CAN6_SG_FCM2_read/1 -> HAL_IN/54
  R_CAN6_FCM3_CAN6_SG_FCM3_read/1 -> HAL_IN/55
  R_CAN6_FCM4_CAN6_SG_FCM4_read/1 -> HAL_IN/56
  R_CAN6_SRR1_CAN6_SG_SRR1_read/1 -> HAL_IN/57
  HAL_IN/1 -> P_BHAL_CAN1_outputs_BHAL_CAN1_outputs_write/1
  HAL_IN/2 -> P_BHAL_CAN2_outputs_BHAL_CAN2_outputs_write/1
  HAL_IN/3 -> P_BHAL_CAN3_outputs_BHAL_CAN3_outputs_write/1
  HAL_IN/4 -> P_BHAL_CAN4_outputs_BHAL_CAN4_outputs_write/1
  HAL_IN/5 -> P_BHAL_CAN5_outputs_BHAL_CAN5_outputs_write/1
  HAL_IN/6 -> P_BHAL_CAN6_outputs_BHAL_CAN6_outputs_write/1

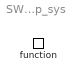
== system SWC_HALIN_type/P_WDGCDD/run_SWC_HALIN_AppCallWDG_StartUp_sys ==
  function : TriggerPort  TriggerType=function-call  IsSimulinkFunction=on  FunctionName=run_SWC_HALIN_AppCallWDG_StartUp  VariantControl=(inherit)

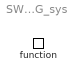
== system SWC_HALIN_type/P_WDGCDD/run_SWC_HALIN_AppCallWDG_sys ==
  function : TriggerPort  TriggerType=function-call  IsSimulinkFunction=on  FunctionName=run_SWC_HALIN_AppCallWDG  VariantControl=(inherit)

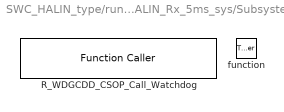
== system SWC_HALIN_type/run_SWC_HALIN_Rx_5ms_sys/Subsystem ==
  function : TriggerPort  TriggerType=function-call  VariantControl=(inherit)
  R_WDGCDD_CSOP_Call_Watchdog : FunctionCaller  FunctionPrototype=R_WDGCDD_CSOP_Call_Watchdog()

== stateflow chart SWC_HALIN_type/run_SWC_HALIN_Rx_5ms_sys/hcu_main_sched ==
  state Main_Scheduler
    (default) -> (junction 31) : {
        |   Sys_Init_done = FALSE;
        |   trig_Read_NVM_00;
        |   trig_ReadIMUOffset_00;
        | }
    Main_Scheduler -> (junction 31) : {Sys_Init_done = TRUE;}
    (junction 31) -> (junction 34) [order 1] : [
        |    Sys_Init_done &&...
        |    !VHAL_FusionSchedReq_flg
        | ]
    (junction 31) -> (junction 38) [order 2]
    (junction 34) -> (junction 36) : {
        |     trig_WDG;
        |     trig_GetNMID;
        |     trig_HAL_IN_10;
        |     trig_GetDID;
        |     trig_HAL_CDD_10_1;
        |     trig_HAL_DKC_10_2;
        |     trig_HAL_DKC_10_3;
        |     trig_INP_20;
        |     trig_APP_30;
        |     trig_OUTP_40;
        |     trig_OUTP_AFTER_40_1;
        |     trig_SetDID;
        |     trig_HAL_OUT_50;
        |     trig_HAL_OUTAFTER_50_1;
        |    }
    (junction 36) -> (junction 38)
  (default) -> Main_Scheduler
  data: VHAL_FusionSchedReq_flg input; Sys_Init_done local double; FALSE parameter; TRUE parameter
  events: trig_Read_NVM_00 output FUNCTION_CALL_EVENT; trig_ReadIMUOffset_00 output FUNCTION_CALL_EVENT; trig_WDG output FUNCTION_CALL_EVENT; trig_GetNMID output FUNCTION_CALL_EVENT; trig_HAL_IN_10 output FUNCTION_CALL_EVENT; trig_GetDID output FUNCTION_CALL_EVENT; trig_HAL_CDD_10_1 output FUNCTION_CALL_EVENT; trig_HAL_DKC_10_2 output FUNCTION_CALL_EVENT; trig_HAL_DKC_10_3 output FUNCTION_CALL_EVENT; trig_INP_20 output FUNCTION_CALL_EVENT; trig_APP_30 output FUNCTION_CALL_EVENT; trig_OUTP_40 output FUNCTION_CALL_EVENT; trig_OUTP_AFTER_40_1 output FUNCTION_CALL_EVENT; trig_SetDID output FUNCTION_CALL_EVENT; trig_HAL_OUT_50 output FUNCTION_CALL_EVENT; trig_HAL_OUTAFTER_50_1 output FUNCTION_CALL_EVENT
